simulink model "sample06c_speed_mode_angle_p_I2C0_and_I2C1"  (R2024b)
settings: Solver=ode1  StartTime=0.0  StopTime=inf  FixedStep=0.005  RelTol=1e-3  EnableMultiTasking=on
libraries: roller485lib x6
settings Model: ExtModeTrigDuration=2  Creator=kawata  LastModifiedBy=kawata
settings SolverCC: AutoInsertRateTranBlk=on
settings DataIOCC: ReturnWorkspaceOutputs=off
settings OptimizationCC: EnhancedBackFolding=on  PassReuseOutputArgsAs=Individual arguments  ZeroExternalMemoryAtStartup=off  ZeroInternalMemoryAtStartup=off  MaxStackSize=64  OptimizeBlockOrder=speed  DifferentSizesBufferReuse=on  OptimizationCustomize=off  EfficientTunableParamExpr=on
settings DebuggingCC: ParameterTunabilityLossMsg=error
settings HardwareCC: ProdBitPerPointer=32  ProdBitPerSizeT=32  ProdBitPerPtrDiffT=32  ProdLargestAtomicInteger=Long  ProdLargestAtomicFloat=Double  ProdWordSize=32  ProdHWDeviceType=ARM Compatible->ARM Cortex  UseEmbeddedCoderFeatures=off  UseSimulinkCoderFeatures=off
settings SFSimCC: MATLABDynamicMemAlloc=off
settings RTWCC: Description=Embedded Coder  SystemTargetFile=ert.tlc  HardwareBoard=Raspberry Pi Pico (Arduino Compatible)  TLCOptions="-aInlineSetEventsForThisBaseRateFcn=TLC_FALSE -aSuppressMultiTaskScheduler=TLC_FALSE   -aRateBasedStepFcn=1"  TemplateMakefile=ert_default_tmf  Toolchain=Arduino ARM RP2040  BuildConfiguration=Faster Runs
settings CodeAppCC: ForceParamTrailComments=on  IgnoreCustomStorageClasses=off  OperatorAnnotations=on  SimulinkDataObjDesc=on  SFDataObjDesc=on  InsertBlockDesc=on
settings ERTTargetCC: SupportContinuousTime=on  SupportNonInlinedSFcns=on  SupportVariableSizeSignals=on  ExtModeTransport=3  ExtModeStaticAlloc=on  ExtModeAutomaticAllocSize=off  ExtModeStaticAllocSize=65536  ExtModeMexFile=ext_xcp  ExtModeIntrfLevel=Level2 - Open  InlinedParameterPlacement=Hierarchical  DynamicArrayContainerType=coder::array

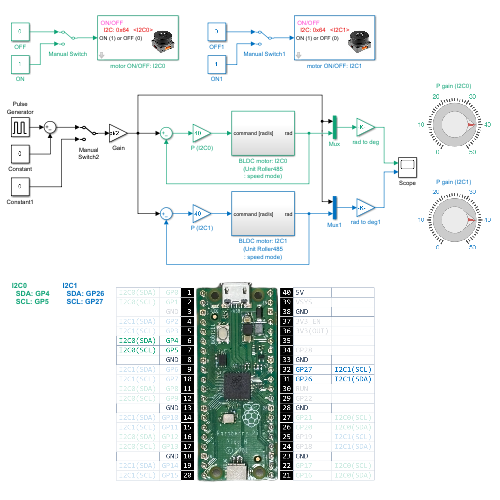
[thumbnail: Simulink's stored preview of the top-level diagram]
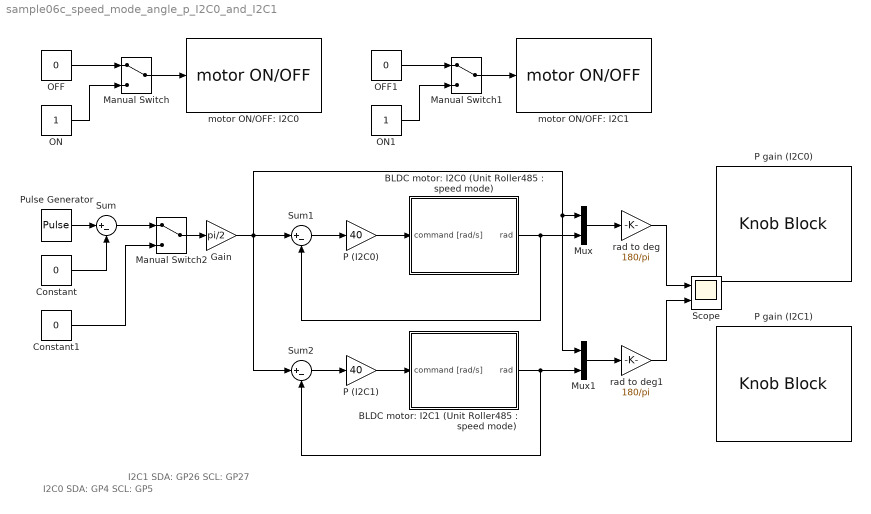
== system sample06c_speed_mode_angle_p_I2C0_and_I2C1 ==
  note: I2C0
      | SDA: GP4
      | SCL: GP5
  note: I2C1
      | SDA: GP26
      | SCL: GP27
  "BLDC motor: I2C0 (Unit Roller485 : speed mode)" : Subsystem
  "BLDC motor: I2C1 (Unit Roller485 : speed mode)" : Subsystem
  Constant : Constant  Value=0
  Constant1 : Constant  Value=0
  Gain : Gain  Gain=pi/2
  Manual Switch2 : ManualSwitch
  Manual Switch : ManualSwitch
  Manual Switch1 : ManualSwitch
  Mux : Mux  Inputs=2
  Mux1 : Mux  Inputs=2
  OFF : Constant  Value=0
  OFF1 : Constant  Value=0
  ON : Constant
  ON1 : Constant
  P (I2C0) : Gain  Gain=40
  P (I2C1) : Gain  Gain=40
  P gain (I2C0) : KnobBlock  LabelPosition=Hide  ScaleMax=50  TickInterval=10
  P gain (I2C1) : KnobBlock  LabelPosition=Hide  ScaleMax=50  TickInterval=10
  Pulse Generator : DiscretePulseGenerator  PulseType=Time based  Period=4  PulseWidth=50  PhaseDelay=1
  Scope : Scope  NumInputPorts=2
  Sum : Sum  Inputs=|+-
  Sum1 : Sum  Inputs=|+-
  Sum2 : Sum  Inputs=|+-
  motor ON/OFF: I2C0 : roller485lib/motor ON//OFF  I2CAddress=0x64  I2CModule=0
      settings: SourceProductName=Roller485 Library
  motor ON/OFF: I2C1 : roller485lib/motor ON//OFF  I2CAddress=0x64  I2CModule=1
      settings: SourceProductName=Roller485 Library
  rad to deg : Gain  Gain=180/pi
  rad to deg1 : Gain  Gain=180/pi
  wires:
  Manual Switch/1 -> motor ON/OFF: I2C0/1
  OFF/1 -> Manual Switch/1
  ON/1 -> Manual Switch/2
  Constant/1 -> Sum/2
  Pulse Generator/1 -> Sum/1
  Mux/1 -> rad to deg/1
  P (I2C0)/1 -> "BLDC motor: I2C0 (Unit Roller485 : speed mode)"/1(command [rad/s])
  Gain/1 -> Sum2/1, Mux1/1, Mux/1, Sum1/1
  "BLDC motor: I2C0 (Unit Roller485 : speed mode)"/1(rad) -> Sum1/2, Mux/2
  Manual Switch2/1 -> Gain/1
  Sum/1 -> Manual Switch2/1
  Constant1/1 -> Manual Switch2/2
  Sum1/1 -> P (I2C0)/1
  Sum2/1 -> P (I2C1)/1
  P (I2C1)/1 -> "BLDC motor: I2C1 (Unit Roller485 : speed mode)"/1(command [rad/s])
  ON1/1 -> Manual Switch1/2
  OFF1/1 -> Manual Switch1/1
  Manual Switch1/1 -> motor ON/OFF: I2C1/1
  Mux1/1 -> rad to deg1/1
  "BLDC motor: I2C1 (Unit Roller485 : speed mode)"/1(rad) -> Mux1/2, Sum2/2
  rad to deg/1 -> Scope/1
  rad to deg1/1 -> Scope/2

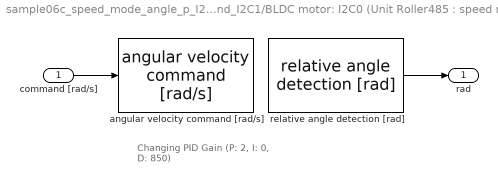
== system sample06c_speed_mode_angle_p_I2C0_and_I2C1/BLDC motor: I2C0 (Unit Roller485 : speed mode) ==
  note: Changing PID Gain
      | (P: 2, I: 0, D: 850)
  command [rad/s] : Inport
  angular velocity command [rad/s] : roller485lib/I2C Write/angular velocity command [rad//s]  I2CAddress=0x64  I2CModule=0  speed_P=2  speed_I=0  speed_D=850  set_time1=0  set_time2=0
      settings: SourceProductName=Roller485 Library
  relative angle detection [rad] : roller485lib/I2C Read/relative angle detection [rad]  I2CAddress=0x64  I2CModule=0  sample_time=-1  set_time=0
      settings: SourceProductName=Roller485 Library
  rad : Outport
  wires:
  command [rad/s]/1 -> angular velocity command [rad/s]/1
  relative angle detection [rad]/1 -> rad/1

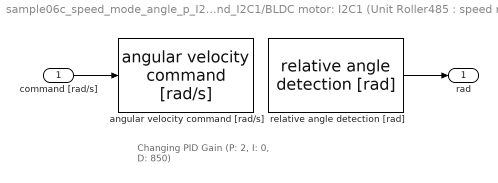
== system sample06c_speed_mode_angle_p_I2C0_and_I2C1/BLDC motor: I2C1 (Unit Roller485 : speed mode) ==
  note: Changing PID Gain
      | (P: 2, I: 0, D: 850)
  command [rad/s] : Inport
  angular velocity command [rad/s] : roller485lib/I2C Write/angular velocity command [rad//s]  I2CAddress=0x64  I2CModule=1  speed_P=2  speed_I=0  speed_D=850  set_time1=0  set_time2=0
      settings: SourceProductName=Roller485 Library
  relative angle detection [rad] : roller485lib/I2C Read/relative angle detection [rad]  I2CAddress=0x64  I2CModule=1  sample_time=-1  set_time=0
      settings: SourceProductName=Roller485 Library
  rad : Outport
  wires:
  relative angle detection [rad]/1 -> rad/1
  command [rad/s]/1 -> angular velocity command [rad/s]/1
